simulink model "Validation_of_PS"  (R2024a)
settings: Solver=ode4  StartTime=0.0  StopTime=inf  FixedStep=0.01  RelTol=1e-6  AbsTol=1e-6
libraries: simulink x1
settings Model: PauseTimes=45  Creator=SPOT  LastModifiedBy=SPOT
settings OptimizationCC: EnhancedBackFolding=on  PassReuseOutputArgsAs=Individual arguments  ZeroExternalMemoryAtStartup=off  ZeroInternalMemoryAtStartup=off  MaxStackSize=64  OptimizeBlockOrder=speed  DifferentSizesBufferReuse=on  OptimizationCustomize=off  EfficientTunableParamExpr=on
settings DebuggingCC: ParameterTunabilityLossMsg=error
settings HardwareCC: ProdBitPerLong=64  ProdLargestAtomicInteger=LongLong  ProdLargestAtomicFloat=Double  ProdLongLongMode=on  ProdHWDeviceType=ARM Compatible->ARM 64-bit (LP64)
settings SFSimCC: MATLABDynamicMemAlloc=off
settings RTWCC: Description=Embedded Coder  SystemTargetFile=ert.tlc  HardwareBoard=NVIDIA Jetson  TLCOptions="-aInlineSetEventsForThisBaseRateFcn=TLC_FALSE -aSuppressMultiTaskScheduler=TLC_FALSE  -aRateBasedStepFcn=0"  TemplateMakefile=ert_default_tmf  TargetLang=C++  GPUComputeCapability=3.5
settings CodeAppCC: ForceParamTrailComments=on  IgnoreCustomStorageClasses=off  OperatorAnnotations=on  SimulinkDataObjDesc=on  SFDataObjDesc=on  InsertBlockDesc=on
settings ERTTargetCC: TargetLangStandard=C++11 (ISO)  MatFileLogging=on  SupportContinuousTime=on  SupportVariableSizeSignals=on

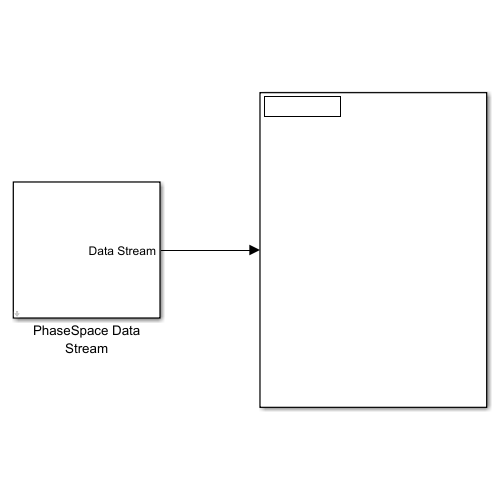
[thumbnail: Simulink's stored preview of the top-level diagram]
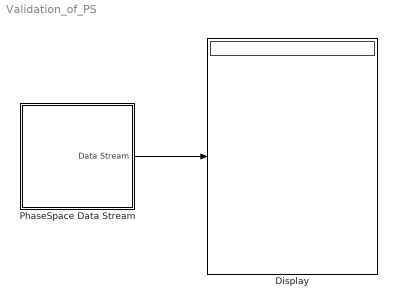
== system Validation_of_PS ==
  Display : Display
  PhaseSpace Data Stream : Subsystem  mask{platformSelection=1}
      mask prompts: platformSelection "Platform Selection"
  wires:
  PhaseSpace Data Stream/1(Data Stream) -> Display/1

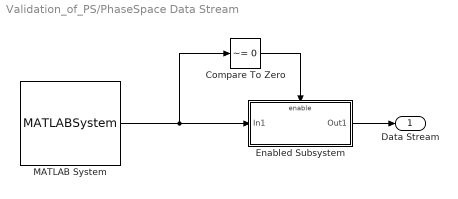
== system Validation_of_PS/PhaseSpace Data Stream ==
  Compare To Zero : simulink/Logic and Bit Operations/Compare To Zero  relop=~=  OutDataTypeStr=boolean
  Enabled Subsystem : Subsystem  TreatAsAtomicUnit=on
  MATLAB System : MATLABSystem  System=PhaseSpace_ALL  platformSelection=platformSelection  sampleRate=0.1  SampleTime=0.01
      mask Type: PhaseSpace_ALL
      mask Display:
      | disp('Stream_PS_ALL');
      | port_label('output',1,'y');
  Data Stream : Outport  VectorParamsAs1DForOutWhenUnconnected=off
  wires:
  MATLAB System/1 -> Enabled Subsystem/1(In1), Compare To Zero/1
  Enabled Subsystem/1(Out1) -> Data Stream/1
  Compare To Zero/1 -> Enabled Subsystem/Enable

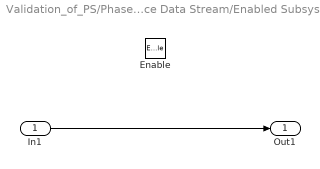
== system Validation_of_PS/PhaseSpace Data Stream/Enabled Subsystem ==
  In1 : Inport
  Enable : EnablePort
  Out1 : Outport  VectorParamsAs1DForOutWhenUnconnected=off
  wires:
  In1/1 -> Out1/1
